simulink model "two_tanks_baseline_dT"  (Simulink 7.5)
settings: Solver=ode45  StartTime=0.0  StopTime=1000  MaxStep=.01  RelTol=1e-3
model workspace (MAT data in the model file):
  x1o : Simulink.Parameter (value not decoded)
  a1 : Simulink.Parameter (value not decoded)
  a2 : Simulink.Parameter (value not decoded)
  A_1 : Simulink.Parameter (value not decoded)
  A_2 : Simulink.Parameter (value not decoded)
  gamma : Simulink.Parameter (value not decoded)
  g : Simulink.Parameter (value not decoded)
  x1_max : Simulink.Parameter (value not decoded)
  x2_max : Simulink.Parameter (value not decoded)
  u_max : Simulink.Parameter (value not decoded)
  Ts : Simulink.Parameter (value not decoded)
  x1f : Simulink.Parameter (value not decoded)
  ku : Simulink.Parameter (value not decoded)
  delta_g : Simulink.Parameter (value not decoded)
settings Model: Creator=Administrator  LastModifiedBy=jporter
settings DebuggingCC: StrictBusMsg=Warning

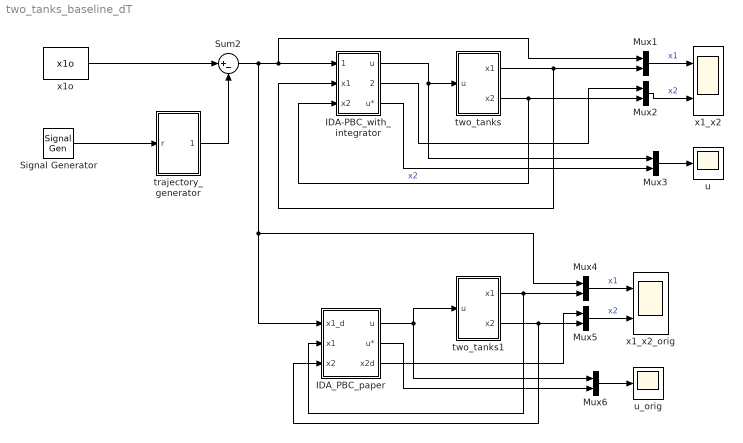
== system two_tanks_baseline_dT ==
  IDA-PBC_with_integrator : Subsystem  mask{k2=4, eps1=.8, eps3=.9, q=10, A_1=A_1, A_2=A_2, a1=a1, a2=a2, gamma=gamma, u_max=u_max, x1_max=x1_max, g=g, Ts=Ts, ku=ku}
      mask prompts: k2 "k2 [0,infty)"; eps1 "eps1 [0,1)"; eps3 "eps3 [0,1)"; q "q > 0"; A_1 "A_1 (cm^2)"; A_2 "A_2 (cm^2)"; a1 "a1 (cm^2)"; a2 "a2 (cm^2)"; g "g (cm/s^2)"; Ts "sample-time [Ts] (seconds)"
      mask init:
      | if k2 < 0
      |     k2 = 1;
      | end
      | if (eps1 >= 1) | (eps1 <= 0)
      |     eps1 = .5;
      | end
      | if (eps3 >= 1) | (eps3 <= 0)
      |     eps3 = .5;
      | end
      | k3 = eps3*4/A_1;
      | k1 = eps1*(4*A_1*k2 - A_1^2*k2*k3)/A_2;
      | E_Qd=eig([-1/(k1*A_1),1/(k2*A_1),0;0,-1/(k2*A_2),0;k3/k1,0,-k3/k1])
      | %p = [k1;-k2*gamma+k1*k2*k3-k2*k3+k2;k1^2]
      | p = [k1;k2*(1-gamma);k1]
      | %cl_num = k2^2*gamma^2 + ((1-k1)*k2^2*k3 - 2*k2^2)*gamma + (k1-1)*k2^2*k3 + k2^2 + k1^3 + k1^2;
      | %cl_den = k2^2*gamma^2 + 2*((1-k1)*k3-1)*k2^2*gamma + (k1^2-2*k1+1)*k2^2*k3^2 + 2*(k1-1)*k2^2*k3 + k2^2 + k1^4 + k1^2;
      | %cl = -cl_num/cl_den
  IDA_PBC_paper : Subsystem  mask{k1=10, mult2=1.01, A_1=A_1, A_2=A_2, a1=a1, a2=a2, gamma=gamma, u_max=u_max, g=g, Ts=Ts}
      mask prompts: mult2 "mult2 >= 1"; gamma "gamma in [0,1]"; g "g (cm/s^2)"
      mask init:
      | if ( k1 < 0 )
      |     k1 = 1.0;
      | end
      | if ( mult2 < 1 )
      |     mult2 = 2;
      | end
      | k2 = mult2 * (A_2/A_1)*(k1 / 4);
      | 
      | K = [k1 (1-gamma)*k2];
      | 
      | A1 = A_1;
      | A2 = A_2;
  Mux{1..6} (6 alike) : Mux  Inputs=2
  Signal Generator : SignalGenerator  WaveForm=square  Amplitude=x1f-x1o  Frequency=1/1000
  Sum2 : Sum  Inputs=|+-  OutDataType=fixdt(1, 16)  OutScaling=2^0
  trajectory_generator : Subsystem  mask{zeta=.9, wn=.05, Ts=Ts}
      mask prompts: zeta "zeta (0 < zeta <= 1)"; wn "wn (radians/sec)"; Ts "Sample Time [Ts] (seconds)"
      mask init:
      | num=[wn^2];
      | den=[1, 2*zeta*wn, wn^2];
      | Hs=tf(num,den);
      | Hz=c2d(Hs,Ts,'tustin');
  two_tanks : Subsystem  mask{x1o=x1o, x2o=x1o*((1-gamma*delta_g)*a1/a2)^2, a1=a1, a2=a2, A_1=A_1, A_2=A_2, gamma=gamma*delta_g, u_max=u_max, x1_max=x1_max, x2_max=x2_max, g=g, ku=ku}
      mask prompts: x1o "x1o (cm)"; x2o "x2o (cm)"; a1 "a1 (cm2)"; a2 "a2 (cm2)"; A_1 "A_1 (cm2)"; A_2 "A_2 (cm2)"; gamma "gamma in [0,1]"; g "g (cm/s2)"
  two_tanks1 : Subsystem  mask{x1o=x1o, x2o=x1o*((1-gamma*delta_g)*a1/a2)^2, a1=a1, a2=a2, A_1=A_1, A_2=A_2, gamma=gamma*delta_g, u_max=u_max, x1_max=x1_max, x2_max=x2_max, g=g, ku=ku}
      mask prompts: x1o "x1o (cm)"; x2o "x2o (cm)"; a1 "a1 (cm2)"; a2 "a2 (cm2)"; A_1 "A_1 (cm2)"; A_2 "A_2 (cm2)"; gamma "gamma in [0,1]"; g "g (cm/s2)"
  u : Scope
      settings: TimeRange=400  YMin=10.25  YMax=14  SaveName=u_new  SampleInput=on  SampleTime=Ts
  u_orig : Scope
      settings: YMin=0  YMax=100  SaveName=u_orig  SampleInput=on  SampleTime=Ts
  x1_x2 : Scope  NumInputPorts=2
      settings: YMin=10~20  YMax=35~70  SaveName=x1_x2_new  SampleInput=on  SampleTime=Ts
  x1_x2_orig : Scope  NumInputPorts=2
      settings: YMin=12.5~20  YMax=30~70  SaveName=x1_x2_orig  SampleInput=on  SampleTime=Ts
  x1o : Constant  Value=x1o  OutDataType=fixdt(1, 16)  OutScaling=2^0  SampleTime=Ts
  wires:
  x1o/1 -> Sum2/1
  Mux1/1 -> x1_x2/1  "x1"
  two_tanks/2(x2) -> IDA-PBC_with_integrator/3(x2), Mux2/2  "x2"
  IDA-PBC_with_integrator/1(u) -> two_tanks/1(u), Mux3/1
  Sum2/1 -> IDA-PBC_with_integrator/1(x1d), Mux1/1, IDA_PBC_paper/1(x1_d), Mux4/1
  two_tanks/1(x1) -> Mux1/2, IDA-PBC_with_integrator/2(x1)
  Mux2/1 -> x1_x2/2  "x2"
  IDA-PBC_with_integrator/2(x2d) -> Mux2/1
  Signal Generator/1 -> trajectory_generator/1(r)
  trajectory_generator/1(r_traj) -> Sum2/2
  Mux3/1 -> u/1
  IDA-PBC_with_integrator/3(u*) -> Mux3/2
  Mux4/1 -> x1_x2_orig/1  "x1"
  Mux5/1 -> x1_x2_orig/2  "x2"
  Mux6/1 -> u_orig/1
  two_tanks1/1(x1) -> Mux4/2, IDA_PBC_paper/2(x1)
  two_tanks1/2(x2) -> Mux5/2, IDA_PBC_paper/3(x2)
  IDA_PBC_paper/1(u) -> two_tanks1/1(u), Mux6/1
  IDA_PBC_paper/2(u*) -> Mux6/2
  IDA_PBC_paper/3(x2d) -> Mux5/1

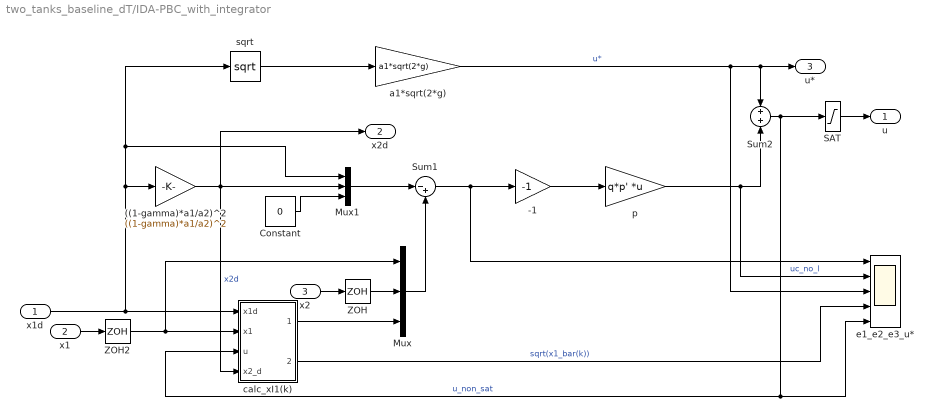
== system two_tanks_baseline_dT/IDA-PBC_with_integrator ==
  x1d : Inport
  x1 : Inport  Port=2
  x2 : Inport  Port=3
  ((1-gamma)*a1/a2)^2 : Gain  Gain=((1-gamma)*a1/a2)^2  ParameterDataType=fixdt(1, 16)  ParameterScaling=2^0  OutDataType=fixdt(1, 16)  OutScaling=2^0
  -1 : Gain  Gain=-1  ParameterDataType=fixdt(1, 16)  ParameterScaling=2^0  OutDataType=fixdt(1, 16)  OutScaling=2^0
  Constant : Constant  Value=0  OutDataType=fixdt(1, 16)  OutScaling=2^0  SampleTime=Ts
  Mux : Mux  Inputs=3
  Mux1 : Mux  Inputs=3
  SAT : Saturate  UpperLimit=u_max  LowerLimit=0  OutDataType=fixdt(1, 16)  OutScaling=2^0
  Sum1 : Sum  Inputs=|-+  OutDataType=fixdt(1, 16)  OutScaling=2^0
  Sum2 : Sum  Priority=-1  OutDataType=fixdt(1, 16)  OutScaling=2^0
  ZOH : ZeroOrderHold  Priority=-2  SampleTime=Ts
  ZOH2 : ZeroOrderHold  Priority=-2  SampleTime=Ts
  a1*sqrt(2*g) : Gain  Gain=a1*sqrt(2*g)  ParameterDataType=fixdt(1, 16)  ParameterScaling=2^0  OutDataType=fixdt(1, 16)  OutScaling=2^0
  calc_xI1(k) : Subsystem  Priority=0
  e1_e2_e3_u* : Scope  NumInputPorts=5
      settings: YMin=-10~-75~10~0~-25  YMax=12.5~75~70~0.75~125  SampleInput=on  SampleTime=.2
  p : Gain  Gain=q*p'  Multiplication=Matrix(K*u)  ParameterDataType=fixdt(1, 16)  ParameterScaling=2^0  OutDataType=fixdt(1, 16)  OutScaling=2^0
  sqrt : Math  Operator=sqrt  OutDataType=fixdt(1, 16)  OutScaling=2^0  SaturateOnIntegerOverflow=on
  u : Outport
  x2d : Outport  Port=2
  u* : Outport  Port=3
  wires:
  x1d/1 -> calc_xI1(k)/1(x1d), sqrt/1, Mux1/1, ((1-gamma)*a1/a2)^2/1
  SAT/1 -> u/1
  sqrt/1 -> a1*sqrt(2*g)/1
  Sum2/1 -> SAT/1, e1_e2_e3_u*/5, calc_xI1(k)/3(u)  "u_non_sat"
  x1/1 -> ZOH2/1
  Mux1/1 -> Sum1/1
  Mux/1 -> Sum1/2
  Sum1/1 -> -1/1, e1_e2_e3_u*/1
  -1/1 -> p/1
  p/1 -> Sum2/2, e1_e2_e3_u*/2  "uc_no_l"
  a1*sqrt(2*g)/1 -> e1_e2_e3_u*/3, Sum2/1, u*/1  "u*"
  Constant/1 -> Mux1/3
  ((1-gamma)*a1/a2)^2/1 -> Mux1/2, x2d/1, calc_xI1(k)/4(x2_d)  "x2d"
  calc_xI1(k)/1(xI1(k)) -> Mux/3
  x2/1 -> ZOH/1
  ZOH/1 -> Mux/2
  ZOH2/1 -> calc_xI1(k)/2(x1), Mux/1
  calc_xI1(k)/2(sqrt(x1 + x1_lin)) -> e1_e2_e3_u*/4  "sqrt(x1_bar(k))"

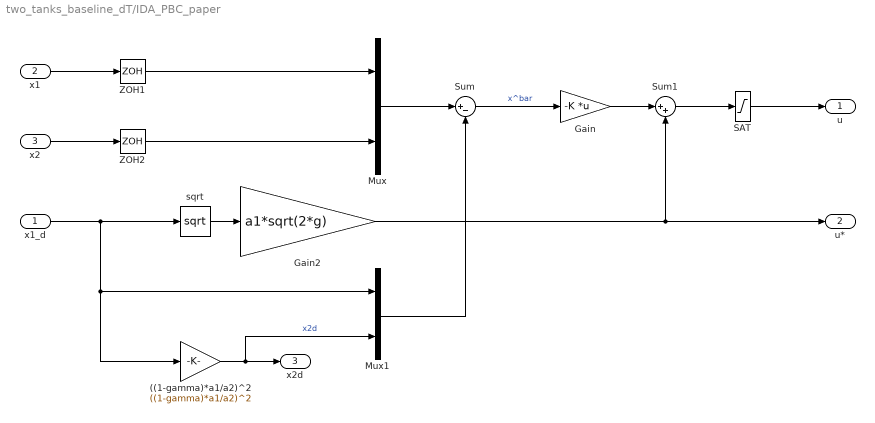
== system two_tanks_baseline_dT/IDA_PBC_paper ==
  x1_d : Inport
  x1 : Inport  Port=2
  x2 : Inport  Port=3
  ((1-gamma)*a1/a2)^2 : Gain  Gain=((1-gamma)*a1/a2)^2  ParameterDataType=fixdt(1, 16)  ParameterScaling=2^0  OutDataType=fixdt(1, 16)  OutScaling=2^0
  Gain : Gain  Gain=-K  Multiplication=Matrix(K*u)  ParameterDataType=fixdt(1, 16)  ParameterScaling=2^0  OutDataType=fixdt(1, 16)  OutScaling=2^0
  Gain2 : Gain  Gain=a1*sqrt(2*g)  ParameterDataType=fixdt(1, 16)  ParameterScaling=2^0  OutDataType=fixdt(1, 16)  OutScaling=2^0
  Mux : Mux  Inputs=2
  Mux1 : Mux  Inputs=2
  SAT : Saturate  UpperLimit=u_max  LowerLimit=0  OutDataType=fixdt(1, 16)  OutScaling=2^0
  Sum : Sum  Inputs=|+-  OutDataType=fixdt(1, 16)  OutScaling=2^0
  Sum1 : Sum  Inputs=|++  OutDataType=fixdt(1, 16)  OutScaling=2^0
  ZOH1 : ZeroOrderHold  Priority=-2  SampleTime=Ts
  ZOH2 : ZeroOrderHold  Priority=-2  SampleTime=Ts
  sqrt : Math  Operator=sqrt  OutDataType=fixdt(1, 16)  OutScaling=2^0  SaturateOnIntegerOverflow=on
  u : Outport
  u* : Outport  Port=2
  x2d : Outport  Port=3
  wires:
  x1/1 -> ZOH1/1
  Mux/1 -> Sum/1
  Sum/1 -> Gain/1  "x^bar"
  Gain/1 -> Sum1/1
  x2/1 -> ZOH2/1
  x1_d/1 -> sqrt/1, Mux1/1, ((1-gamma)*a1/a2)^2/1
  Mux1/1 -> Sum/2
  sqrt/1 -> Gain2/1
  Gain2/1 -> u*/1, Sum1/2
  Sum1/1 -> SAT/1
  ((1-gamma)*a1/a2)^2/1 -> x2d/1, Mux1/2  "x2d"
  SAT/1 -> u/1
  ZOH2/1 -> Mux/2
  ZOH1/1 -> Mux/1

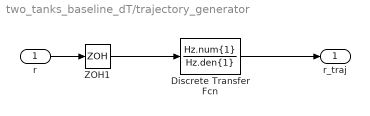
== system two_tanks_baseline_dT/trajectory_generator ==
  r : Inport
  Discrete Transfer Fcn : DiscreteTransferFcn  Numerator=Hz.num{1}  Denominator=Hz.den{1}  SampleTime=-1
  ZOH1 : ZeroOrderHold  Priority=-2  SampleTime=Ts
  r_traj : Outport
  wires:
  r/1 -> ZOH1/1
  Discrete Transfer Fcn/1 -> r_traj/1
  ZOH1/1 -> Discrete Transfer Fcn/1

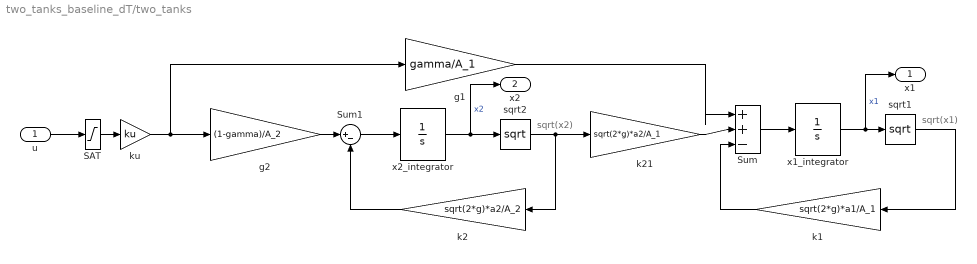
== system two_tanks_baseline_dT/two_tanks ==
  note: sqrt(x1)
  note: sqrt(x2)
  u : Inport  OutDataType=fixdt(1, 16)  OutScaling=2^0
  SAT : Saturate  UpperLimit=u_max  LowerLimit=0  OutDataType=fixdt(1, 16)  OutScaling=2^0
  Sum : Sum  Inputs=|++-  OutDataType=fixdt(1, 16)  OutScaling=2^0
  Sum1 : Sum  Inputs=|+-  OutDataType=fixdt(1, 16)  OutScaling=2^0
  g1 : Gain  Gain=gamma/A_1  ParameterDataType=fixdt(1, 16)  ParameterScaling=2^0  OutDataType=fixdt(1, 16)  OutScaling=2^0
  g2 : Gain  Gain=(1-gamma)/A_2  ParameterDataType=fixdt(1, 16)  ParameterScaling=2^0  OutDataType=fixdt(1, 16)  OutScaling=2^0
  k1 : Gain  Gain=sqrt(2*g)*a1/A_1  ParameterDataType=fixdt(1, 16)  ParameterScaling=2^0  OutDataType=fixdt(1, 16)  OutScaling=2^0
  k2 : Gain  Gain=sqrt(2*g)*a2/A_2  ParameterDataType=fixdt(1, 16)  ParameterScaling=2^0  OutDataType=fixdt(1, 16)  OutScaling=2^0
  k21 : Gain  Gain=sqrt(2*g)*a2/A_1  ParameterDataType=fixdt(1, 16)  ParameterScaling=2^0  OutDataType=fixdt(1, 16)  OutScaling=2^0
  ku : Gain  Gain=ku  ParameterDataType=fixdt(1, 16)  ParameterScaling=2^0  OutDataType=fixdt(1, 16)  OutScaling=2^0
  sqrt1 : Math  Operator=sqrt  OutDataType=fixdt(1, 16)  OutScaling=2^0  SaturateOnIntegerOverflow=on
  sqrt2 : Math  Operator=sqrt  OutDataType=fixdt(1, 16)  OutScaling=2^0  SaturateOnIntegerOverflow=on
  x1_integrator : Integrator  InitialCondition=x1o  LimitOutput=on  UpperSaturationLimit=x1_max  LowerSaturationLimit=0
  x2_integrator : Integrator  InitialCondition=x2o  LimitOutput=on  UpperSaturationLimit=x2_max  LowerSaturationLimit=0
  x1 : Outport  OutDataType=fixdt(1, 16)  OutScaling=2^0
  x2 : Outport  Port=2  OutDataType=fixdt(1, 16)  OutScaling=2^0
  wires:
  Sum/1 -> x1_integrator/1
  k1/1 -> Sum/3
  sqrt1/1 -> k1/1
  sqrt2/1 -> k2/1, k21/1
  x2_integrator/1 -> sqrt2/1, x2/1  "x2"
  k2/1 -> Sum1/2
  Sum1/1 -> x2_integrator/1
  k21/1 -> Sum/2
  g2/1 -> Sum1/1
  x1_integrator/1 -> sqrt1/1, x1/1  "x1"
  u/1 -> SAT/1
  g1/1 -> Sum/1
  SAT/1 -> ku/1
  ku/1 -> g2/1, g1/1

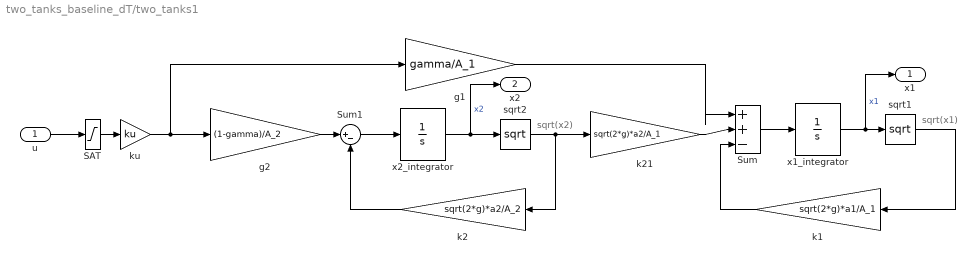
== system two_tanks_baseline_dT/two_tanks1 ==
  note: sqrt(x1)
  note: sqrt(x2)
  u : Inport  OutDataType=fixdt(1, 16)  OutScaling=2^0
  SAT : Saturate  UpperLimit=u_max  LowerLimit=0  OutDataType=fixdt(1, 16)  OutScaling=2^0
  Sum : Sum  Inputs=|++-  OutDataType=fixdt(1, 16)  OutScaling=2^0
  Sum1 : Sum  Inputs=|+-  OutDataType=fixdt(1, 16)  OutScaling=2^0
  g1 : Gain  Gain=gamma/A_1  ParameterDataType=fixdt(1, 16)  ParameterScaling=2^0  OutDataType=fixdt(1, 16)  OutScaling=2^0
  g2 : Gain  Gain=(1-gamma)/A_2  ParameterDataType=fixdt(1, 16)  ParameterScaling=2^0  OutDataType=fixdt(1, 16)  OutScaling=2^0
  k1 : Gain  Gain=sqrt(2*g)*a1/A_1  ParameterDataType=fixdt(1, 16)  ParameterScaling=2^0  OutDataType=fixdt(1, 16)  OutScaling=2^0
  k2 : Gain  Gain=sqrt(2*g)*a2/A_2  ParameterDataType=fixdt(1, 16)  ParameterScaling=2^0  OutDataType=fixdt(1, 16)  OutScaling=2^0
  k21 : Gain  Gain=sqrt(2*g)*a2/A_1  ParameterDataType=fixdt(1, 16)  ParameterScaling=2^0  OutDataType=fixdt(1, 16)  OutScaling=2^0
  ku : Gain  Gain=ku  ParameterDataType=fixdt(1, 16)  ParameterScaling=2^0  OutDataType=fixdt(1, 16)  OutScaling=2^0
  sqrt1 : Math  Operator=sqrt  OutDataType=fixdt(1, 16)  OutScaling=2^0  SaturateOnIntegerOverflow=on
  sqrt2 : Math  Operator=sqrt  OutDataType=fixdt(1, 16)  OutScaling=2^0  SaturateOnIntegerOverflow=on
  x1_integrator : Integrator  InitialCondition=x1o  LimitOutput=on  UpperSaturationLimit=x1_max  LowerSaturationLimit=0
  x2_integrator : Integrator  InitialCondition=x2o  LimitOutput=on  UpperSaturationLimit=x2_max  LowerSaturationLimit=0
  x1 : Outport  OutDataType=fixdt(1, 16)  OutScaling=2^0
  x2 : Outport  Port=2  OutDataType=fixdt(1, 16)  OutScaling=2^0
  wires:
  Sum/1 -> x1_integrator/1
  k1/1 -> Sum/3
  sqrt1/1 -> k1/1
  sqrt2/1 -> k2/1, k21/1
  x2_integrator/1 -> sqrt2/1, x2/1  "x2"
  k2/1 -> Sum1/2
  Sum1/1 -> x2_integrator/1
  k21/1 -> Sum/2
  g2/1 -> Sum1/1
  x1_integrator/1 -> sqrt1/1, x1/1  "x1"
  u/1 -> SAT/1
  g1/1 -> Sum/1
  SAT/1 -> ku/1
  ku/1 -> g2/1, g1/1

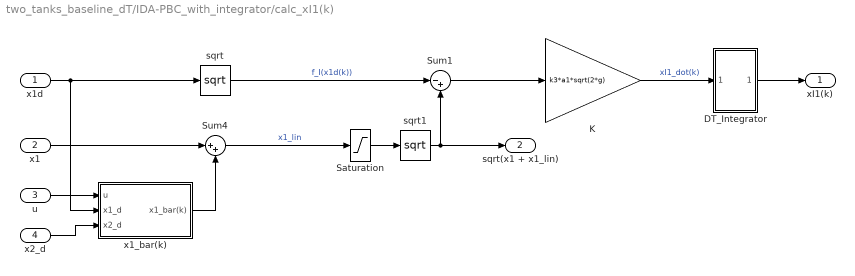
== system two_tanks_baseline_dT/IDA-PBC_with_integrator/calc_xI1(k) ==
  x1d : Inport
  x1 : Inport  Port=2
  u : Inport  Port=3
  x2_d : Inport  Port=4
  DT_Integrator : Subsystem
  K : Gain  Gain=k3*a1*sqrt(2*g)  ParameterDataType=fixdt(1, 16)  ParameterScaling=2^0  OutDataType=fixdt(1, 16)  OutScaling=2^0
  Saturation : Saturate  UpperLimit=x1_max  LowerLimit=0  OutDataType=fixdt(1, 16)  OutScaling=2^0
  Sum1 : Sum  Inputs=|-+  OutDataType=fixdt(1, 16)  OutScaling=2^0
  Sum4 : Sum  Inputs=|++  OutDataType=fixdt(1, 16)  OutScaling=2^0
  sqrt : Math  Operator=sqrt  OutDataType=fixdt(1, 16)  OutScaling=2^0  SaturateOnIntegerOverflow=on
  sqrt1 : Math  Operator=sqrt  OutDataType=fixdt(1, 16)  OutScaling=2^0  SaturateOnIntegerOverflow=on
  x1_bar(k) : Subsystem
  xI1(k) : Outport
  sqrt(x1 + x1_lin) : Outport  Port=2
  wires:
  x1d/1 -> sqrt/1, x1_bar(k)/2(x1_d)
  sqrt/1 -> Sum1/1  "f_I(x1d(k))"
  x1_bar(k)/1(x1_bar(k)) -> Sum4/2
  u/1 -> x1_bar(k)/1(u)
  Sum4/1 -> Saturation/1  "x1_lin"
  Sum1/1 -> K/1
  K/1 -> DT_Integrator/1(In1)  "xI1_dot(k)"
  DT_Integrator/1(Out1) -> xI1(k)/1
  x2_d/1 -> x1_bar(k)/3(x2_d)
  x1/1 -> Sum4/1
  Saturation/1 -> sqrt1/1
  sqrt1/1 -> Sum1/2, sqrt(x1 + x1_lin)/1

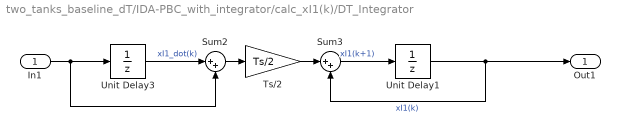
== system two_tanks_baseline_dT/IDA-PBC_with_integrator/calc_xI1(k)/DT_Integrator ==
  In1 : Inport
  Sum2 : Sum  Inputs=|++  OutDataType=fixdt(1, 16)  OutScaling=2^0
  Sum3 : Sum  Inputs=|++  OutDataType=fixdt(1, 16)  OutScaling=2^0
  Ts/2 : Gain  Gain=Ts/2  ParameterDataType=fixdt(1, 16)  ParameterScaling=2^0  OutDataType=fixdt(1, 16)  OutScaling=2^0
  Unit Delay1 : UnitDelay  SampleTime=-1
  Unit Delay3 : UnitDelay  SampleTime=-1
  Out1 : Outport
  wires:
  In1/1 -> Sum2/2, Unit Delay3/1
  Unit Delay3/1 -> Sum2/1  "xI1_dot(k)"
  Sum2/1 -> Ts/2/1
  Sum3/1 -> Unit Delay1/1  "xI1(k+1)"
  Ts/2/1 -> Sum3/1
  Unit Delay1/1 -> Sum3/2, Out1/1  "xI1(k)"

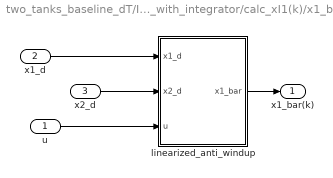
== system two_tanks_baseline_dT/IDA-PBC_with_integrator/calc_xI1(k)/x1_bar(k) ==
  u : Inport
  x1_d : Inport  Port=2
  x2_d : Inport  Port=3
  linearized_anti_windup : Subsystem
  x1_bar(k) : Outport
  wires:
  linearized_anti_windup/1(x1_bar) -> x1_bar(k)/1
  u/1 -> linearized_anti_windup/3(u)
  x1_d/1 -> linearized_anti_windup/1(x1_d)
  x2_d/1 -> linearized_anti_windup/2(x2_d)

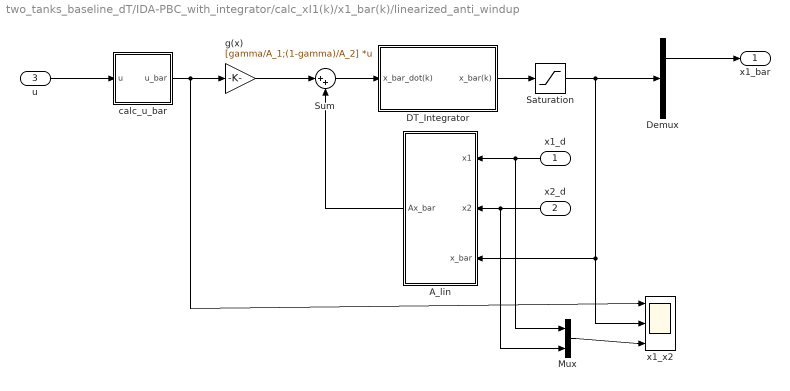
== system two_tanks_baseline_dT/IDA-PBC_with_integrator/calc_xI1(k)/x1_bar(k)/linearized_anti_windup ==
  x1_d : Inport
  x2_d : Inport  Port=2
  u : Inport  Port=3
  A_lin : Stateflow chart  TreatAsAtomicUnit=on
  DT_Integrator : Subsystem
  Demux : Demux  Outputs=2
  Mux : Mux  Inputs=2
  Saturation : Saturate  UpperLimit=[x1_max,x2_max]  LowerLimit=-[x1_max,x2_max]  OutDataType=fixdt(1, 16)  OutScaling=2^0
  Sum : Sum  Inputs=|++  OutDataType=fixdt(1, 16)  OutScaling=2^0
  calc_u_bar : Subsystem
  g(x) : Gain  Gain=[gamma/A_1;(1-gamma)/A_2]  Multiplication=Matrix(K*u)  ParameterDataType=fixdt(1, 16)  ParameterScaling=2^0  OutDataType=fixdt(1, 16)  OutScaling=2^0
  x1_x2 : Scope  NumInputPorts=3
      settings: YMin=-200~-80~0  YMax=25~20~55  SaveName=x1_x2_new1  SampleInput=on  SampleTime=.5
  x1_bar : Outport
  wires:
  g(x)/1 -> Sum/1
  u/1 -> calc_u_bar/1(u)
  calc_u_bar/1(u_bar) -> g(x)/1, x1_x2/1
  A_lin/1(Ax_bar) -> Sum/2
  x2_d/1 -> A_lin/2(x2), Mux/2
  x1_d/1 -> A_lin/1(x1), Mux/1
  Sum/1 -> DT_Integrator/1(x_bar_dot(k))
  Demux/1 -> x1_bar/1
  DT_Integrator/1(x_bar(k)) -> Saturation/1
  Mux/1 -> x1_x2/3
  Saturation/1 -> Demux/1, A_lin/3(x_bar), x1_x2/2

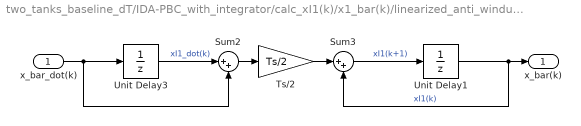
== system two_tanks_baseline_dT/IDA-PBC_with_integrator/calc_xI1(k)/x1_bar(k)/linearized_anti_windup/DT_Integrator ==
  x_bar_dot(k) : Inport
  Sum2 : Sum  Inputs=|++  OutDataType=fixdt(1, 16)  OutScaling=2^0
  Sum3 : Sum  Inputs=|++  OutDataType=fixdt(1, 16)  OutScaling=2^0
  Ts/2 : Gain  Gain=Ts/2  ParameterDataType=fixdt(1, 16)  ParameterScaling=2^0  OutDataType=fixdt(1, 16)  OutScaling=2^0
  Unit Delay1 : UnitDelay  SampleTime=Ts
  Unit Delay3 : UnitDelay  SampleTime=Ts
  x_bar(k) : Outport
  wires:
  x_bar_dot(k)/1 -> Sum2/2, Unit Delay3/1
  Unit Delay3/1 -> Sum2/1  "xI1_dot(k)"
  Sum2/1 -> Ts/2/1
  Sum3/1 -> Unit Delay1/1  "xI1(k+1)"
  Unit Delay1/1 -> Sum3/2, x_bar(k)/1  "xI1(k)"
  Ts/2/1 -> Sum3/1

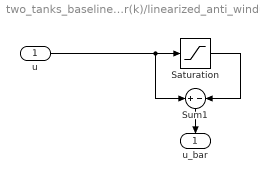
== system two_tanks_baseline_dT/IDA-PBC_with_integrator/calc_xI1(k)/x1_bar(k)/linearized_anti_windup/calc_u_bar ==
  u : Inport
  Saturation : Saturate  UpperLimit=u_max  LowerLimit=0  OutDataType=fixdt(1, 16)  OutScaling=2^0
  Sum1 : Sum  Inputs=+-  OutDataType=fixdt(1, 16)  OutScaling=2^0
  u_bar : Outport
  wires:
  Sum1/1 -> u_bar/1
  u/1 -> Sum1/1, Saturation/1
  Saturation/1 -> Sum1/2

== matlab function IDA-PBC_with_integrator/calc_xI1(k)/x1_bar(k)/linearized_anti_windup/A_lin ==
  settings: updateMethod=DISCRETE  sampleTime=Ts
  data: x1 input double; x2 input double; x_bar input double size=[2]; Ax_bar output double; g parameter double; a1 parameter double; a2 parameter double; A_1 parameter double; A_2 parameter double
function Ax_bar  = fcn(x1, x2, x_bar, g, a1, a2, A_1, A_2)
x_min = 1;
if x1 < x_min
    x1 = x_min;
end
if x2 < x_min
    x2 = x_min;
end
A =[-a1/(A_1*sqrt(x1)), a2/(A_1*sqrt(x2));
0, -a2/(A_2*sqrt(x2))];
A = (1/2)*sqrt(2*g)*A;
Ax_bar = A*x_bar;
